simulink model "Valvula"  (Simulink 8.5)
settings: Solver=ode3  StartTime=0.0  StopTime=1000  RelTol=1e-3
values from neighbouring files (symbols this model uses):
  Fh0 = 0.8946    [TP1.m]
settings Model: Creator=Marcelo  LastModifiedBy=GISP
settings SolverCC: ShapePreserveControl=EnableAll
settings DataIOCC: LimitDataPoints=off  SaveOutput=off  SaveTime=off
settings OptimizationCC: BooleanDataType=off
settings DebuggingCC: SaveWithParameterizedLinksMsg=none  SignalResolutionControl=TryResolveAllWithWarning  MultiTaskDSMMsg=warning  MultiTaskCondExecSysMsg=none  FcnCallInpInsideContextMsg=UseLocalSettings  StrictBusMsg=None
settings HardwareCC: TargetUnknown=on

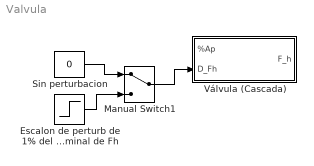
== system Valvula ==
  Escalon de perturb de 1% del valor nominal de Fh : Step  Time=100  After=Fh0*0.01  SampleTime=0
  Manual Switch1 : ManualSwitch
  Sin perturbacion : Constant  Value=0
  Válvula (Cascada) : Subsystem
  wires:
  Manual Switch1/1 -> Válvula (Cascada)/2(D_Fh)
  Sin perturbacion/1 -> Manual Switch1/1
  Escalon de perturb de 1% del valor nominal de Fh/1 -> Manual Switch1/2

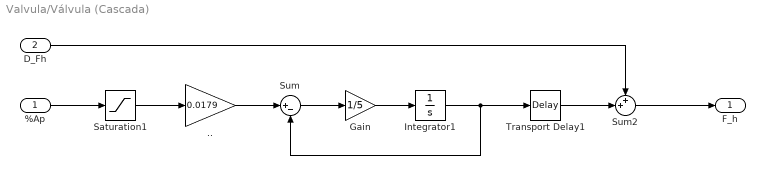
== system Valvula/Válvula (Cascada) ==
  %Ap : Inport
  D_Fh : Inport  Port=2
  .. : Gain  Gain=0.0179
  Gain : Gain  Gain=1/5
  Integrator1 : Integrator  InitialCondition=Fh0
  Saturation1 : Saturate  UpperLimit=100  LowerLimit=0
  Sum : Sum  Inputs=|+-
  Sum2 : Sum  Inputs=++|
  Transport Delay1 : TransportDelay  InitialOutput=Fh0
  F_h : Outport
  wires:
  D_Fh/1 -> Sum2/1
  Sum2/1 -> F_h/1
  %Ap/1 -> Saturation1/1
  Saturation1/1 -> ../1
  Sum/1 -> Gain/1
  Gain/1 -> Integrator1/1
  Integrator1/1 -> Transport Delay1/1, Sum/2
  ../1 -> Sum/1
  Transport Delay1/1 -> Sum2/2
